simulink library "ctransform"  (R2021b)
settings: Solver=VariableStepAuto  StartTime=0.0  StopTime=10.0  RelTol=1e-3
undefined symbols (not defined in the file or in its folder): i, OM, om, theta0
settings Model: Creator=Davide  LastModifiedBy=Davide

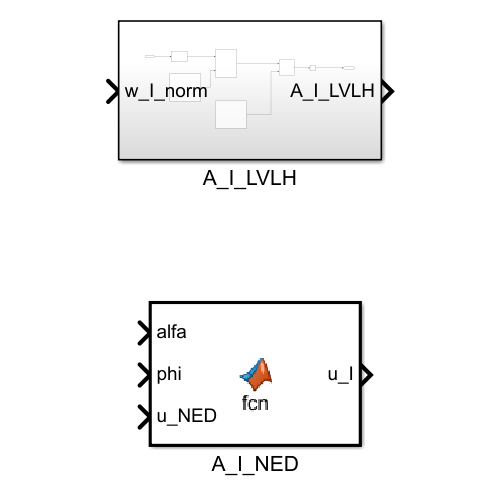
[thumbnail: Simulink's stored preview of the top-level diagram]
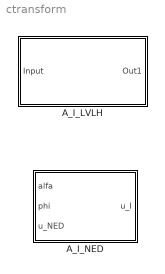
== system ctransform ==
  A_I_LVLH : Subsystem
  A_I_NED : MATLAB Function  TreatAsAtomicUnit=on

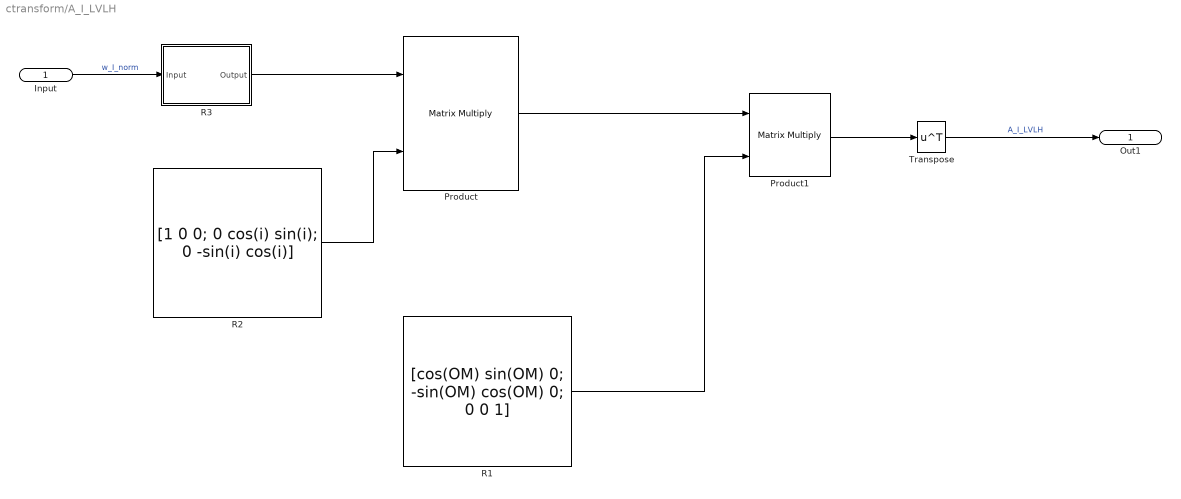
== system ctransform/A_I_LVLH ==
  Input : Inport
  Product : Product  Multiplication=Matrix(*)
  Product1 : Product  Multiplication=Matrix(*)
  R1 : Constant  Value="[cos(OM)  sin(OM) 0; -sin(OM) cos(OM) 0; 0 0 1]"
  R2 : Constant  Value=[1 0 0; 0 cos(i) sin(i); 0 -sin(i) cos(i)]
  R3 : Subsystem
  Transpose : Math  Operator=transpose  SaturateOnIntegerOverflow=on
  Out1 : Outport
  wires:
  Transpose/1 -> Out1/1  "A_I_LVLH"
  Product/1 -> Product1/1
  R2/1 -> Product/2
  Input/1 -> R3/1(Input)  "w_I_norm"
  Product1/1 -> Transpose/1
  R1/1 -> Product1/2
  R3/1(Output) -> Product/1

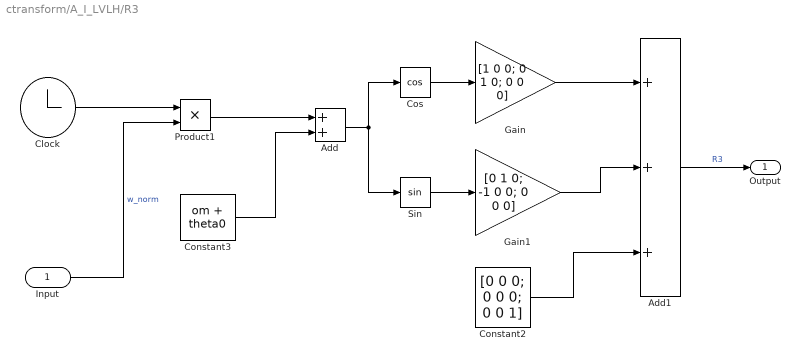
== system ctransform/A_I_LVLH/R3 ==
  Input : Inport
  Add : Sum
  Add1 : Sum  Inputs=+++
  Clock : Clock
  Constant2 : Constant  Value=[0 0 0; 0 0 0; 0 0 1]
  Constant3 : Constant  Value=om + theta0
  Cos : Trigonometry  Operator=cos
  Gain : Gain  Gain=[1 0 0; 0 1 0; 0 0 0]
  Gain1 : Gain  Gain=[0 1 0; -1 0 0; 0 0 0]
  Product1 : Product
  Sin : Trigonometry
  Output : Outport
  wires:
  Clock/1 -> Product1/1
  Product1/1 -> Add/1
  Gain/1 -> Add1/1
  Add1/1 -> Output/1  "R3"
  Add/1 -> Cos/1, Sin/1
  Gain1/1 -> Add1/2
  Cos/1 -> Gain/1
  Constant3/1 -> Add/2
  Sin/1 -> Gain1/1
  Input/1 -> Product1/2  "w_norm"
  Constant2/1 -> Add1/3

== matlab function ctransform/A_I_NED ==
  data: alfa input; u_I output; phi input; u_NED input
function u_I = fcn(alfa,phi,u_NED)
Ar = [cos(alfa), sin(alfa) 0; -sin(alfa) cos(alfa) 0; 0 0 1]*[cos(phi+pi/2) 0 sin(phi+pi/2); 0 1 0; -sin(phi+pi/2) 0 cos(phi+pi/2)];
u_I = Ar'*u_NED;
